simulink model "pruebaj2"  (R2017a)
settings: Solver=ode4  StartTime=0.0  StopTime=10  FixedStep=1e-4  RelTol=1e-3
InitFcn:
  | SimulinkInit
settings Model: Creator=carma  LastModifiedBy=Administrador
settings OptimizationCC: DefaultParameterBehavior=Inlined  PassReuseOutputArgsAs=Individual arguments
settings DebuggingCC: ParameterTunabilityLossMsg=error
settings SFSimCC: MATLABDynamicMemAlloc=off
settings RTWCC: SystemTargetFile=ert.tlc  TemplateMakefile=ert_default_tmf  Description=Embedded Coder  GenerateReport=on  IncludeHyperlinkInReport=on  LaunchReport=on  GenerateTraceInfo=on  GenerateTraceReport=on  GenerateTraceReportSl=on  GenerateTraceReportSf=on  GenerateTraceReportEml=on
settings CodeAppCC: ForceParamTrailComments=on  IgnoreCustomStorageClasses=off  OperatorAnnotations=on  SimulinkDataObjDesc=on  SFDataObjDesc=on  MATLABFcnDesc=on  InsertBlockDesc=on  MATLABSourceComments=on
settings ERTTargetCC: TargetLangStandard=C99 (ISO)  GenerateSampleERTMain=on  SupportContinuousTime=on  InlinedParameterPlacement=NonHierarchical  ERTCustomFileTemplate=example_file_process.tlc

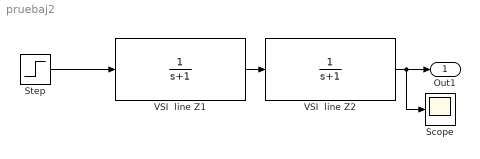
== system pruebaj2 ==
  Scope : Scope
  Step : Step  Time=0  SampleTime=0
  VSI  line Z1 : TransferFcn  Denominator=[1 1]
  VSI  line Z2 : TransferFcn  Denominator=[1 1]
  Out1 : Outport
  wires:
  VSI  line Z1/1 -> VSI  line Z2/1
  Step/1 -> VSI  line Z1/1
  VSI  line Z2/1 -> Scope/1, Out1/1
